simulink model "rfxnl"  (Simulink 4.00)
settings: Solver=ode4  SolverMode=SingleTasking  StartTime=0.0  StopTime=2  FixedStep=.0005  MaxStep=0.0005  MinStep=0.0005  RelTol=1e-3  AbsTol=1e-3
libraries: simulink3 x1
settings Model: LastModifiedBy=arthur  SaveTime=off  SaveOutput=off

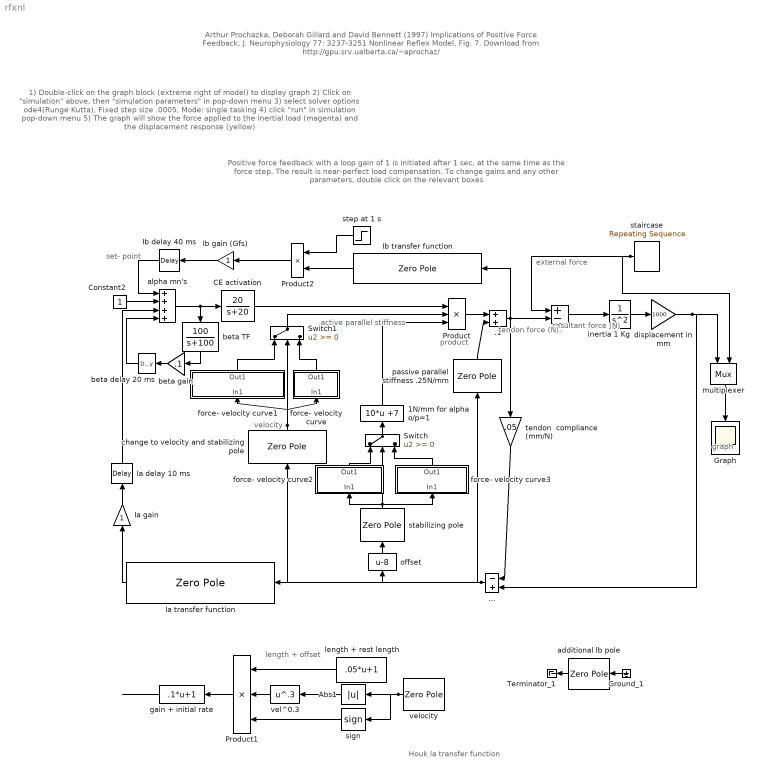
== system rfxnl ==
  note: external
      | force
  note: graph
  note: resultant
      | force
      | (N)
  note: tendon
      | force
      | (N)
  note: product
  note: velocity
  note: active
      | parallel
      | stiffness
  note: set-
      | point
  note: Arthur Prochazka, Deborah Gillard and David Bennett (1997)
      | Implications of Positive Force Feedback,  J. Neurophysiology 77: 3237-3251
      | Nonlinear Reflex Model, Fig. 7.
      | Download from http://gpu.srv.ualberta.ca/~aprochaz/
  note: 1) Double-click on the graph block (extreme right of model) to display graph
      | 2) Click on "simulation" above, then "simulation parameters" in pop-down menu
      | 3) select solver options ode4(Runge Kutta), Fixed step size .0005, Mode: single tasking
      | 4) click "run" in simulation pop-down menu
      | 5) The graph will show the force applied to the inertial load (magenta) and the displacement response (yellow)
  note: Positive force feedback with a loop gain of 1 is initiated after 1 sec, at the same time as the force step.
      | The result is near-perfect load compensation.  To change gains and any other parameters, double click on the relevant boxes
  note: Houk la transfer function
  note: length + offset
  .. : Sum  Inputs=+-  SaturateOnIntegerOverflow=on
  ... : Sum  Orientation=left  Inputs=-+  SaturateOnIntegerOverflow=on
  .1 : Sum  Inputs=++  SaturateOnIntegerOverflow=on
  1N/mm for alpha o/p=1 : Fcn  Orientation=up  Expr=10*u +7
  Abs1 : Abs  Orientation=left  SaturateOnIntegerOverflow=on
  CE activation : TransferFcn  Numerator=[20]  Denominator=[1 20]  AbsoluteTolerance=auto  Realization=auto
  Constant2 : Constant  Value=1
  Graph : Scope
      settings: Orientation=down  TimeRange=2  YMin=0  YMax=30  SaveToWorkspace=off  SaveName=ScopeData  DataFormat=Array  LimitDataPoints=on  MaxDataPoints=5000
  Ground_1 : Ground  Orientation=left
  Ia delay 10 ms : TransportDelay  Orientation=up  DelayTime=.01  InitialInput=0  BufferSize=1024  PadeOrder=0
  Ia gain : Gain  Orientation=up  Gain=1  Multiplication=Element-wise(K.*u)  SaturateOnIntegerOverflow=on
  Ia transfer function : ZeroPole  Orientation=left  Zeros=[0; -.4; -4; -44]  Poles=[-.04; -.8; -1000; -1000]  Gain=[100]  AbsoluteTolerance=auto
  Ib delay 40 ms : TransportDelay  Orientation=left  DelayTime=0.04  InitialInput=0  BufferSize=1024  PadeOrder=0
  Ib gain (Gfs) : Gain  Orientation=left  Gain=1  Multiplication=Element-wise(K.*u)  SaturateOnIntegerOverflow=on
  Ib transfer function : ZeroPole  Orientation=left  Zeros=[-.15; -1.5; -16]  Poles=[-.2; -2; -37]  Gain=[.28]  AbsoluteTolerance=auto
  Product : Product  Inputs=3  Multiplication=Element-wise(.*)  SaturateOnIntegerOverflow=on
  Product1 : Product  Orientation=left  Inputs=3  Multiplication=Element-wise(.*)  SaturateOnIntegerOverflow=on
  Product2 : Product  Orientation=left  Inputs=2  Multiplication=Element-wise(.*)  SaturateOnIntegerOverflow=on
  Switch : Switch  Orientation=up  Threshold=0
  Switch1 : Switch  Orientation=up  Threshold=0
  Terminator_1 : Terminator
  additional lb pole : ZeroPole  Orientation=left  Zeros=[]  Poles=[-33]  Gain=[33]  AbsoluteTolerance=auto
  alpha mn's : Sum  Inputs=++++  SaturateOnIntegerOverflow=on
  beta delay 20 ms : TransportDelay  Orientation=left  DelayTime=.02  InitialInput=0  BufferSize=1024  PadeOrder=0
  beta TF : TransferFcn  Orientation=down  Numerator=[100]  Denominator=[1 100]  AbsoluteTolerance=auto  Realization=auto
  beta gain : Gain  Orientation=left  Gain=.1  Multiplication=Element-wise(K.*u)  SaturateOnIntegerOverflow=on
  change to velocity and stabilizing pole : ZeroPole  Orientation=up  Zeros=[0]  Poles=[-500;-500]  Gain=[1500]  AbsoluteTolerance=auto
  displacement in mm : Gain  Gain=1000  Multiplication=Element-wise(K.*u)  SaturateOnIntegerOverflow=on
  force- velocity curve : Subsystem  Orientation=up
      settings: RTWFcnNameOpts=Auto  RTWFileNameOpts=Auto
      mask Display: disp('1/(1-u)')
  force- velocity curve1 : Subsystem  Orientation=up
      settings: RTWFcnNameOpts=Auto  RTWFileNameOpts=Auto
      mask Display: disp('1+.5(1-exp(-1.5u))')
  force- velocity curve2 : Subsystem  Orientation=up
      settings: RTWFcnNameOpts=Auto  RTWFileNameOpts=Auto
      mask Display: disp('1-exp(-.15u)')
  force- velocity curve3 : Subsystem  Orientation=up
      settings: RTWFcnNameOpts=Auto  RTWFileNameOpts=Auto
      mask Display: disp('-1+exp(.15u)')
  gain + initial rate : Fcn  Orientation=left  Expr=.1*u+1
  inertia 1 Kg : TransferFcn  Numerator=[1]  Denominator=[1 0 0]  AbsoluteTolerance=auto  Realization=auto
  length + rest length : Fcn  Orientation=left  Expr=.05*u+1
  multiplexer : Mux  Orientation=down  Inputs=2
      settings: DisplayOption=none
  offset : Fcn  Orientation=up  Expr=u-8
  passive parallel stiffness .25N/mm : ZeroPole  Orientation=up  Zeros=[-25]  Poles=[-500]  Gain=[5]  AbsoluteTolerance=auto
  sign : Signum  Orientation=left
  stabilizing pole : ZeroPole  Orientation=up  Zeros=[ ]  Poles=[-500]  Gain=[500]  AbsoluteTolerance=auto
  staircase : simulink3/Sources/Repeating Sequence  Orientation=left  rep_seq_t=[0 0 1 1 2]  rep_seq_y=[0 10 10 20 20]
  step at 1 s : Step  Orientation=left  Time=1  Before=0  After=1  SampleTime=-1
  tendon  compliance (mm/N) : Gain  Orientation=down  Gain=.05  Multiplication=Element-wise(K.*u)  SaturateOnIntegerOverflow=on
  vel^0.3 : Fcn  Orientation=left  Expr=u^.3
  "velocity " : ZeroPole  Orientation=left  Zeros=[0;]  Poles=[-100;]  Gain=[100]  AbsoluteTolerance=auto
  wires:
  ../1 -> inertia 1 Kg/1
  Ib gain (Gfs)/1 -> Ib delay 40 ms/1
  alpha mn's/1 -> CE activation/1, beta TF/1
  Ib delay 40 ms/1 -> alpha mn's/1
  beta gain/1 -> beta delay 20 ms/1
  Ia transfer function/1 -> Ia gain/1
  .1/1 -> ../2, Ib transfer function/1, tendon  compliance (mm/N)/1
  .../1 -> Ia transfer function/1, offset/1, passive parallel stiffness .25N/mm/1, change to velocity and stabilizing pole/1
  Product/1 -> .1/1
  CE activation/1 -> Product/1
  beta delay 20 ms/1 -> alpha mn's/4
  Ia delay 10 ms/1 -> alpha mn's/3
  Constant2/1 -> alpha mn's/2
  Ib transfer function/1 -> Product2/2
  Product2/1 -> Ib gain (Gfs)/1
  passive parallel stiffness .25N/mm/1 -> .1/2
  offset/1 -> stabilizing pole/1
  beta TF/1 -> beta gain/1
  tendon  compliance (mm/N)/1 -> .../1
  Switch/1 -> 1N/mm for alpha o/p=1/1
  Switch1/1 -> Product/2
  step at 1 s/1 -> Product2/1
  change to velocity and stabilizing pole/1 -> Switch1/2, force- velocity curve1/1(In1), force- velocity curve/1(In1)
  1N/mm for alpha o/p=1/1 -> Product/3
  stabilizing pole/1 -> Switch/2, force- velocity curve2/1(In1), force- velocity curve3/1(In1)
  force- velocity curve1/1(Out1) -> Switch1/1
  displacement in mm/1 -> multiplexer/1, .../2
  staircase/1 -> ../1, multiplexer/2
  force- velocity curve3/1(Out1) -> Switch/3
  force- velocity curve2/1(Out1) -> Switch/1
  force- velocity curve/1(Out1) -> Switch1/3
  multiplexer/1 -> Graph/1
  Ground_1/1 -> additional lb pole/1
  additional lb pole/1 -> Terminator_1/1
  Product1/1 -> gain + initial rate/1
  vel^0.3/1 -> Product1/2
  length + rest length/1 -> Product1/1
  sign/1 -> Product1/3
  Abs1/1 -> vel^0.3/1
  "velocity "/1 -> Abs1/1, sign/1
  ? -> "velocity "/1, length + rest length/1
  gain + initial rate/1 -> ?
  Ia gain/1 -> Ia delay 10 ms/1
  inertia 1 Kg/1 -> displacement in mm/1

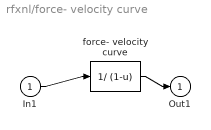
== system rfxnl/force- velocity curve ==
  In1 : Inport  Port=1  LatchInput=off
  force- velocity curve : Fcn  Expr=1/ (1-u)
  Out1 : Outport  Port=1
  wires:
  In1/1 -> force- velocity curve/1
  force- velocity curve/1 -> Out1/1

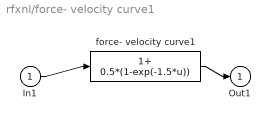
== system rfxnl/force- velocity curve1 ==
  In1 : Inport  Port=1  LatchInput=off
  force- velocity curve1 : Fcn  Expr=1+ 0.5*(1-exp(-1.5*u))
  Out1 : Outport  Port=1
  wires:
  In1/1 -> force- velocity curve1/1
  force- velocity curve1/1 -> Out1/1

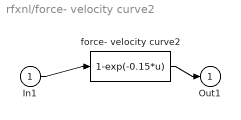
== system rfxnl/force- velocity curve2 ==
  In1 : Inport  Port=1  LatchInput=off
  force- velocity curve2 : Fcn  Expr=1-exp(-0.15*u)
  Out1 : Outport  Port=1
  wires:
  In1/1 -> force- velocity curve2/1
  force- velocity curve2/1 -> Out1/1

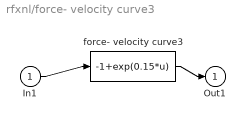
== system rfxnl/force- velocity curve3 ==
  In1 : Inport  Port=1  LatchInput=off
  force- velocity curve3 : Fcn  Expr=-1+exp(0.15*u)
  Out1 : Outport  Port=1
  wires:
  In1/1 -> force- velocity curve3/1
  force- velocity curve3/1 -> Out1/1
